simulink model "WT_FirstModel_2020"  (R2020b)
settings: Solver=FixedStepAuto  StartTime=0.0  StopTime=60  FixedStep=0.1  RelTol=1e-3
undefined symbols (not defined in the file): a, b, g, H, K_F, K_R, l, m, R, t_F, t_R, V, W, Z_RF, Z_RR
settings Model: Creator=emilybeeler  LastModifiedBy=mluser

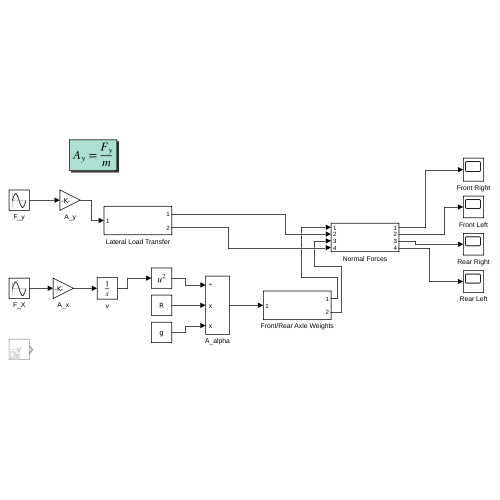
[thumbnail: Simulink's stored preview of the top-level diagram]
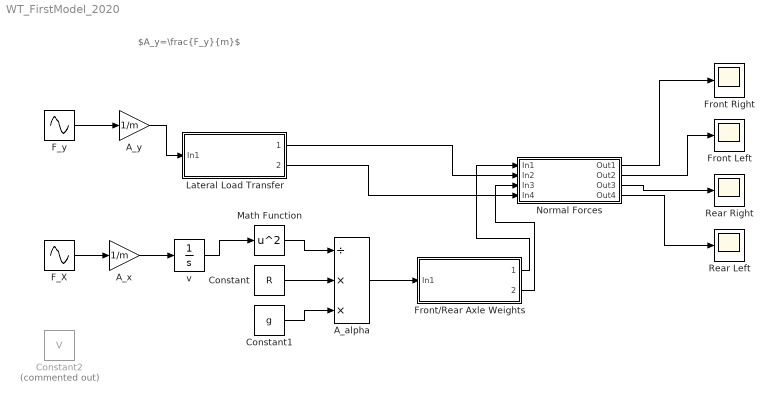
== system WT_FirstModel_2020 ==
  note: $A_y=\frac{F_y}{m}$
  A_alpha : Product  Inputs=/**
  A_x : Gain  Gain=1/m
  A_y : Gain  Gain=1/m
  Constant : Constant  Value=R
  Constant1 : Constant  Value=g
  Constant2 : Constant  Commented=on  Value=V
  F_X : Sin  Amplitude=500  Frequency=.2  SampleTime=0
  F_y : Sin  Amplitude=50  Frequency=.2  SampleTime=0
  Front Left : Scope
  Front Right : Scope
  Front/Rear Axle Weights : Subsystem
  Lateral Load Transfer : Subsystem
  Math Function : Math  Operator=square  SaturateOnIntegerOverflow=on
  Normal Forces : Subsystem
  Rear Left : Scope
  Rear Right : Scope
  v : Integrator  InitialCondition=100
  wires:
  Math Function/1 -> A_alpha/1
  Constant/1 -> A_alpha/2
  Constant1/1 -> A_alpha/3
  A_alpha/1 -> Front/Rear Axle Weights/1(In1)
  Lateral Load Transfer/1(1) -> Normal Forces/2(In2)
  Lateral Load Transfer/2(2) -> Normal Forces/4(In4)
  Front/Rear Axle Weights/1(1) -> Normal Forces/1(In1)
  Front/Rear Axle Weights/2(2) -> Normal Forces/3(In3)
  Normal Forces/1(Out1) -> Front Right/1
  Normal Forces/2(Out2) -> Front Left/1
  Normal Forces/3(Out3) -> Rear Right/1
  Normal Forces/4(Out4) -> Rear Left/1
  A_y/1 -> Lateral Load Transfer/1(In1)
  F_y/1 -> A_y/1
  F_X/1 -> A_x/1
  A_x/1 -> v/1
  v/1 -> Math Function/1

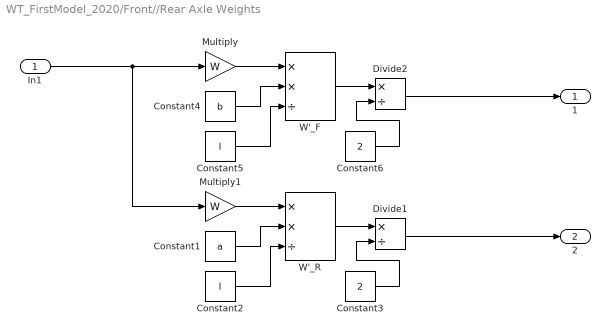
== system WT_FirstModel_2020/Front//Rear Axle Weights ==
  In1 : Inport
  Constant1 : Constant  Value=a
  Constant2 : Constant  Value=l
  Constant3 : Constant  Value=2
  Constant4 : Constant  Value=b
  Constant5 : Constant  Value=l
  Constant6 : Constant  Value=2
  Divide1 : Product  Inputs=*/
  Divide2 : Product  Inputs=*/
  Multiply : Gain  Gain=W
  Multiply1 : Gain  Gain=W
  W'_F : Product  Inputs=**/
  W'_R : Product  Inputs=**/
  1 : Outport
  2 : Outport  Port=2
  wires:
  Multiply/1 -> W'_F/1
  Constant5/1 -> W'_F/3
  Constant6/1 -> Divide2/2
  Constant4/1 -> W'_F/2
  W'_F/1 -> Divide2/1
  In1/1 -> Multiply1/1, Multiply/1
  Multiply1/1 -> W'_R/1
  Constant2/1 -> W'_R/3
  Constant3/1 -> Divide1/2
  Constant1/1 -> W'_R/2
  W'_R/1 -> Divide1/1
  Divide2/1 -> 1/1
  Divide1/1 -> 2/1

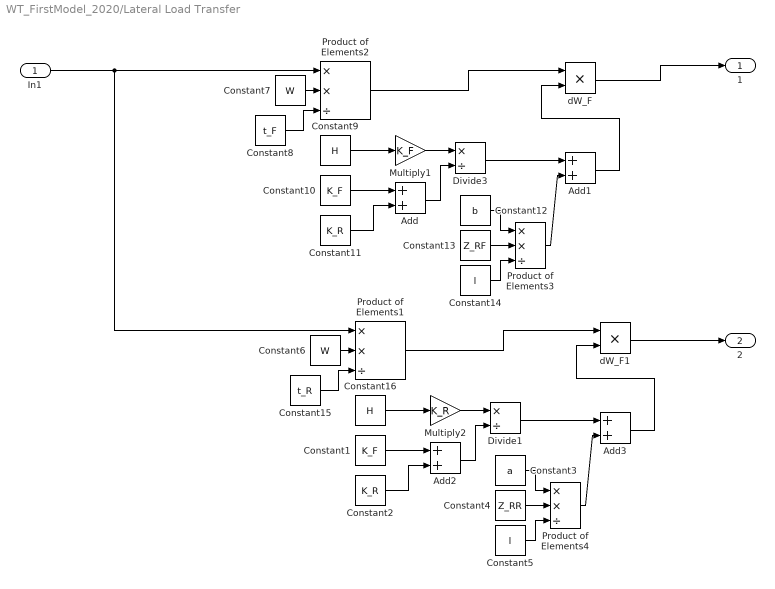
== system WT_FirstModel_2020/Lateral Load Transfer ==
  In1 : Inport
  Add{,1..3} (4 alike) : Sum
  Constant1 : Constant  Value=K_F
  Constant10 : Constant  Value=K_F
  Constant11 : Constant  Value=K_R
  Constant12 : Constant  Value=b
  Constant13 : Constant  Value=Z_RF
  Constant14 : Constant  Value=l
  Constant15 : Constant  Value=t_R
  Constant16 : Constant  Value=H
  Constant2 : Constant  Value=K_R
  Constant3 : Constant  Value=a
  Constant4 : Constant  Value=Z_RR
  Constant5 : Constant  Value=l
  Constant6 : Constant  Value=W
  Constant7 : Constant  Value=W
  Constant8 : Constant  Value=t_F
  Constant9 : Constant  Value=H
  Divide1 : Product  Inputs=*/
  Divide3 : Product  Inputs=*/
  Multiply1 : Gain  Gain=K_F
  Multiply2 : Gain  Gain=K_R
  Product of Elements{1..4} (4 alike) : Product  Inputs=**/
  dW_F : Product  Inputs=**
  dW_F1 : Product  Inputs=**
  1 : Outport
  2 : Outport  Port=2
  wires:
  In1/1 -> Product of Elements1/1, Product of Elements2/1
  Constant11/1 -> Add/2
  Divide3/1 -> Add1/1
  Add1/1 -> dW_F/2
  Constant7/1 -> Product of Elements2/2
  Product of Elements2/1 -> dW_F/1
  Constant8/1 -> Product of Elements2/3
  Multiply1/1 -> Divide3/1
  Add/1 -> Divide3/2
  Constant13/1 -> Product of Elements3/2
  Constant14/1 -> Product of Elements3/3
  Constant12/1 -> Product of Elements3/1
  Constant9/1 -> Multiply1/1
  Constant10/1 -> Add/1
  Product of Elements3/1 -> Add1/2
  dW_F/1 -> 1/1
  Constant2/1 -> Add2/2
  Divide1/1 -> Add3/1
  Add3/1 -> dW_F1/2
  Constant6/1 -> Product of Elements1/2
  Product of Elements1/1 -> dW_F1/1
  Constant15/1 -> Product of Elements1/3
  Multiply2/1 -> Divide1/1
  Add2/1 -> Divide1/2
  Constant4/1 -> Product of Elements4/2
  Constant5/1 -> Product of Elements4/3
  Constant3/1 -> Product of Elements4/1
  Constant16/1 -> Multiply2/1
  Constant1/1 -> Add2/1
  Product of Elements4/1 -> Add3/2
  dW_F1/1 -> 2/1

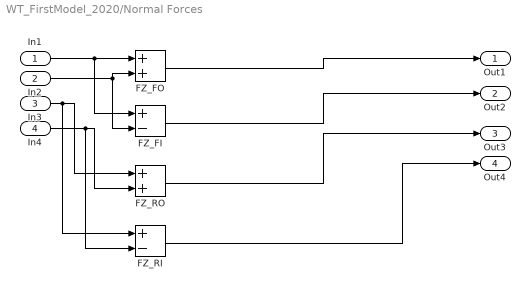
== system WT_FirstModel_2020/Normal Forces ==
  In1 : Inport
  In2 : Inport  Port=2
  In3 : Inport  Port=3
  In4 : Inport  Port=4
  FZ_FI : Sum  Inputs=+-
  FZ_FO : Sum
  FZ_RI : Sum  Inputs=+-
  FZ_RO : Sum
  Out1 : Outport
  Out2 : Outport  Port=2
  Out3 : Outport  Port=3
  Out4 : Outport  Port=4
  wires:
  In1/1 -> FZ_FI/1, FZ_FO/1
  In2/1 -> FZ_FI/2, FZ_FO/2
  FZ_FI/1 -> Out2/1
  In3/1 -> FZ_RI/1, FZ_RO/1
  In4/1 -> FZ_RI/2, FZ_RO/2
  FZ_RO/1 -> Out3/1
  FZ_RI/1 -> Out4/1
  FZ_FO/1 -> Out1/1
